simulink model "DC_Motor_Load_PID_block_position_unit_response"  (R2015a)
settings: Solver=ode45  StartTime=0.0  StopTime=10.0  RelTol=1e-3
values from neighbouring files (symbols this model uses):
  BL = B_roller + B_material    (= 0)    [dc_motor_show_data_last.m]    (also in dc_motor_show_data_last_pos.m)
  Bt = Bm + BL    (= 0.0158)    [dc_motor_show_data_last.m]    (also in dc_motor_show_data_last_pos.m = 0.00093)
  JL = J_roller + J_material    (= 0.000102958)    [dc_motor_show_data_last.m]    (also in dc_motor_show_data_last_pos.m)
  Jt = Jm + JL    (= 0.002622958)    [dc_motor_show_data_last.m]    (also in dc_motor_show_data_last_pos.m = 0.000155558)
  Kd = Kp*Td    (= 8.33268608414)    [ZIEGLER_NICHOLCUS_METHOD_tuning_pid.m]    (also in dc_motor_show_data.m = 0.0189; dc_motor_show_data_PID_range_errors_show.m = 0.09; dc_motor_show_data_PID_range_response.m = 0.09; dc_motor_show_data_PID_test_ST.m = 0.09)
  Ke = 0.1    [DC_MOTOR.m]    (also in ZIEGLER_NICHOLCUS_METHOD_tuning_pid.m = 0.57; dc_motor_show_data.m = 0.57; dc_motor_show_data_PID_range_errors_show.m; dc_motor_show_data_PID_range_response.m)
  Ki = Kp/Ti    (= 21.5184713376)    [ZIEGLER_NICHOLCUS_METHOD_tuning_pid.m]    (also in dc_motor_show_data.m = 39.9; dc_motor_show_data_PID_range_errors_show.m = 2.98; dc_motor_show_data_PID_range_response.m = 2.98; dc_motor_show_data_PID_test_ST.m = 2.98)
  Kp = 0.2*K_cr    (= 16.4)    [ZIEGLER_NICHOLCUS_METHOD_tuning_pid.m]    (also in dc_motor_show_data.m = 2.1398; dc_motor_show_data_PID_range_errors_show.m = 1.25; dc_motor_show_data_PID_range_response.m = 1.25; dc_motor_show_data_PID_test_ST.m = 1.25)
  Kt = 0.2    [DC_MOTOR.m]    (also in ZIEGLER_NICHOLCUS_METHOD_tuning_pid.m = 0.259; dc_motor_show_data.m = 0.259; dc_motor_show_data_PID_range_errors_show.m; dc_motor_show_data_PID_range_response.m)
  La = 0.143    [dc_motor_show_data_last.m]    (also in dc_motor_show_data_last_pos.m = 0.0006)
  r = 0.005    [dc_motor_show_data_last.m]    (also in dc_motor_show_data_last_pos.m)
  Ra = 9.375    [dc_motor_show_data_last.m]    (also in dc_motor_show_data_last_pos.m)
  TL = 0.0017    [dc_motor_show_data_last.m]    (also in dc_motor_show_data_last_pos.m)
libraries: simulink x1
settings Model: Creator=Alfa maSR  LastModifiedBy=Alfa maSR

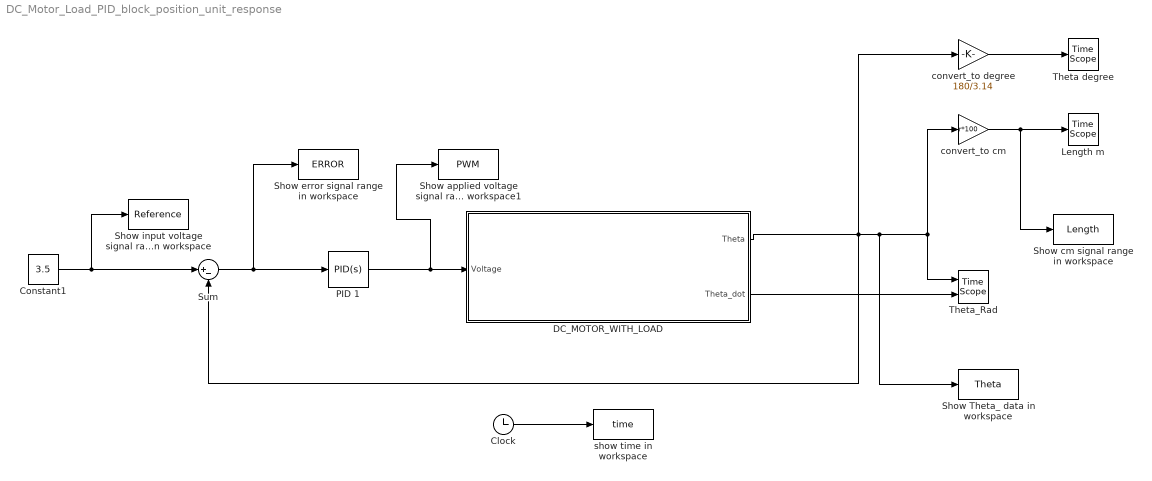
== system DC_Motor_Load_PID_block_position_unit_response ==
  Clock : Clock
  Constant1 : Constant  Value=3.5
  DC_MOTOR_WITH_LOAD : Subsystem
  Length m : TimeScope  DefaultConfigurationName=spbscopes.TimeScopeBlockCfg
  PID 1 : simulink/Continuous/PID Controller  Controller=PID  TimeDomain=Continuous-time  SampleTime=-1  IntegratorMethod=Forward Euler  FilterMethod=Forward Euler  Form=Parallel  UseFilter=on  ControllerParametersSource=internal  P=Kp  I=Ki  D=Kd  N=34.1724449135492  InitialConditionSource=internal  InitialConditionForIntegrator=0  InitialConditionForFilter=0  ExternalReset=none  LimitOutput=off  UpperSaturationLimit=inf  LowerSaturationLimit=-inf  LinearizeAsGain=on  AntiWindupMode=none  Kb=1  TrackingMode=off  Kt=1  PParamMin=[]  PParamMax=[]  IParamMin=[]  IParamMax=[]  DParamMin=[]  DParamMax=[]  NParamMin=[]  NParamMax=[]  KbParamMin=[]  KbParamMax=[]  KtParamMin=[]  KtParamMax=[]  POutMin=[]  POutMax=[]  IOutMin=[]  IOutMax=[]  DOutMin=[]  DOutMax=[]  NOutMin=[]  NOutMax=[]  KbOutMin=[]  KbOutMax=[]  KtOutMin=[]  KtOutMax=[]  IntegratorOutMin=[]  IntegratorOutMax=[]  FilterOutMin=[]  FilterOutMax=[]  SumOutMin=[]  SumOutMax=[]  SumI1OutMin=[]  SumI1OutMax=[]  SumI2OutMin=[]  SumI2OutMax=[]  SumI3OutMin=[]  SumI3OutMax=[]  SumDOutMin=[]  SumDOutMax=[]  SaturationOutMin=[]  SaturationOutMax=[]  IntegratorContinuousStateAttributes=''  IntegratorStateMustResolveToSignalObject=off  IntegratorRTWStateStorageClass=Auto  FilterContinuousStateAttributes=''  FilterStateMustResolveToSignalObject=off  FilterRTWStateStorageClass=Auto  DifferentiatorICPrevScaledInput=0  DifferentiatorOutMin=[]  DifferentiatorOutMax=[]
  Show Theta_ data in workspace : ToWorkspace  VariableName=Theta  SaveFormat=Timeseries  SampleTime=-1
  Show applied voltage signal range in workspace1 : ToWorkspace  VariableName=PWM  SaveFormat=Timeseries  SampleTime=-1
  Show cm signal range in workspace : ToWorkspace  VariableName=Length  SaveFormat=Timeseries  SampleTime=-1
  Show error signal range in workspace : ToWorkspace  VariableName=ERROR  SaveFormat=Timeseries  SampleTime=-1
  Show input voltage signal range in workspace : ToWorkspace  VariableName=Reference  SaveFormat=Timeseries  SampleTime=-1
  Sum : Sum  Inputs=|+-
  Theta degree : TimeScope  DefaultConfigurationName=spbscopes.TimeScopeBlockCfg
  Theta_Rad : TimeScope  DefaultConfigurationName=spbscopes.TimeScopeBlockCfg  NumInputPorts=2
  convert_to cm : Gain  Gain=r*100
  convert_to degree : Gain  Gain=180/3.14
  show time in workspace : ToWorkspace  VariableName=time  SaveFormat=Timeseries  SampleTime=-1
  wires:
  PID 1/1 -> Show applied voltage signal range in workspace1/1, DC_MOTOR_WITH_LOAD/1(Voltage)
  Clock/1 -> show time in workspace/1
  Constant1/1 -> Sum/1, Show input voltage signal range in workspace/1
  Sum/1 -> PID 1/1, Show error signal range in workspace/1
  convert_to cm/1 -> Show cm signal range in workspace/1, Length m/1
  DC_MOTOR_WITH_LOAD/1(Theta) -> Sum/2, convert_to degree/1, Show Theta_ data in workspace/1, convert_to cm/1, Theta_Rad/1
  DC_MOTOR_WITH_LOAD/2(Theta_dot) -> Theta_Rad/2
  convert_to degree/1 -> Theta degree/1

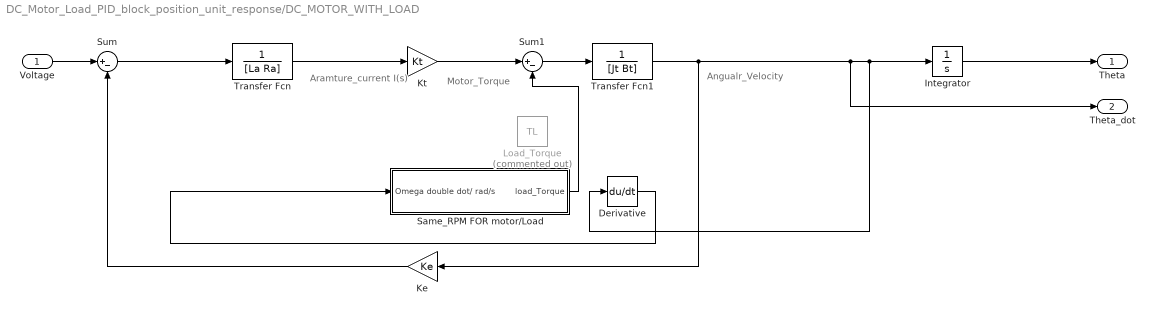
== system DC_Motor_Load_PID_block_position_unit_response/DC_MOTOR_WITH_LOAD ==
  note: Angualr_Velocity
  note: Motor_Torque
  note: Aramture_current
      |           I(s)
  Voltage : Inport
  Derivative : Derivative
  Integrator : Integrator
  Ke : Gain  Gain=Ke
  Kt : Gain  Gain=Kt
  Load_Torque : Constant  Commented=on  Value=TL
  Same_RPM FOR motor/Load : Subsystem
  Sum : Sum  Inputs=|+-
  Sum1 : Sum  Inputs=|+-
  Transfer Fcn : TransferFcn  Denominator=[La Ra]
  Transfer Fcn1 : TransferFcn  Denominator=[Jt Bt]
  Theta : Outport
  Theta_dot : Outport  Port=2
  wires:
  Ke/1 -> Sum/2
  Sum1/1 -> Transfer Fcn1/1
  Sum/1 -> Transfer Fcn/1
  Transfer Fcn/1 -> Kt/1
  Kt/1 -> Sum1/1
  Voltage/1 -> Sum/1
  Derivative/1 -> Same_RPM FOR motor/Load/1(Omega double dot/ rad/s)
  Same_RPM FOR motor/Load/1(load_Torque) -> Sum1/2
  Integrator/1 -> Theta/1
  Transfer Fcn1/1 -> Theta_dot/1, Derivative/1, Integrator/1, Ke/1

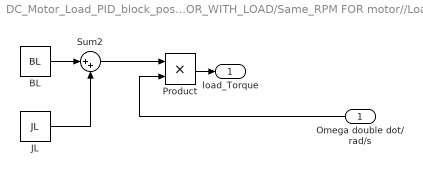
== system DC_Motor_Load_PID_block_position_unit_response/DC_MOTOR_WITH_LOAD/Same_RPM FOR motor//Load ==
  Omega double dot/ rad/s : Inport
  BL : Constant  Value=BL
  JL : Constant  Value=JL
  Product : Product
  Sum2 : Sum  Inputs=|++
  load_Torque : Outport
  wires:
  JL/1 -> Sum2/2
  Omega double dot/ rad/s/1 -> Product/2
  Product/1 -> load_Torque/1
  BL/1 -> Sum2/1
  Sum2/1 -> Product/1
